simulink model "symmetric_lht"  (R2020a)
settings: Solver=FixedStepDiscrete  StartTime=0.0  StopTime=inf  RelTol=1e-3
values from neighbouring files (symbols this model uses):
  fs = fclk(1)*1e6    [setupSystem.m]
  height = heightName(nameIdx)    [setupSystem.m]
  inarray = uint8(simDirNew)    [setupSystem.m]
  nRho = maxRho*2    [setupSystem.m]
  nTheta = length(theta)    [setupSystem.m]
  theta = 0:1:179    [SymmetricLHT.m]    (also in setupSystem.m = (0:1:179))
  width = widthName(nameIdx)    [setupSystem.m]
undefined symbols (not defined in the file or in its folder): rhoBits, rhoMax
libraries: hdlsllib x35, simulink x25, dspsrcs4 x1
(part 1 of 2)
settings Model: DataTypeOverride=Off  SimulationMode=rapid-accelerator  Creator=david  LastModifiedBy=david
settings OptimizationCC: BlockReduction=off  ConditionallyExecuteInputs=off  DefaultParameterBehavior=Inlined
settings DebuggingCC: AlgebraicLoopMsg=error  SingleTaskRateTransMsg=error
settings HardwareCC: ProdBitPerPointer=32  ProdBitPerSizeT=32  ProdBitPerPtrDiffT=32  ProdLargestAtomicFloat=None  ProdIntDivRoundTo=Undefined  ProdEndianess=Unspecified  ProdWordSize=32  ProdHWDeviceType=ASIC/FPGA->ASIC/FPGA  TargetBitPerPointer=64  TargetBitPerSizeT=64  TargetBitPerPtrDiffT=64  TargetLongLongMode=on  TargetIntDivRoundTo=Zero  TargetEndianess=LittleEndian  TargetWordSize=64  TargetHWDeviceType=Custom Processor->MATLAB Host Computer  ProdEqTarget=off

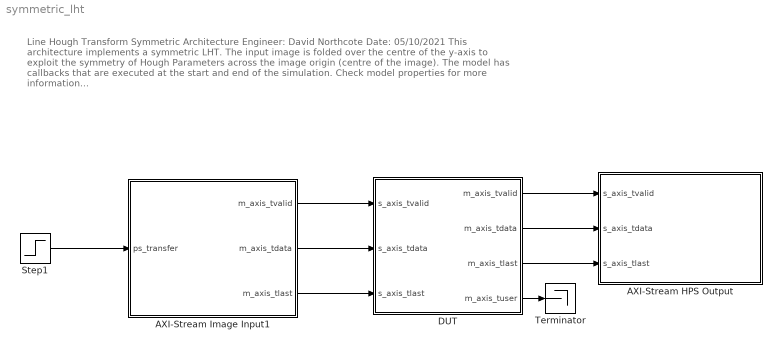
== system symmetric_lht ==
  note: Line Hough Transform Symmetric Architecture
      |
      | Engineer: David Northcote
      | Date: 05/10/2021
      |
      | This architecture implements a symmetric LHT. The input image is folded over the centre of the y-axis to exploit the symmetry of Hough Parameters across the image origin (centre of the image).
      | The model has callbacks that are executed at the start and end of the simulation. Check model properties for more information...
  AXI-Stream HPS Output : Subsystem  mask{height=nRho, width=nTheta, clk=1/fs, d=0}
      mask prompts: height "Image Height:"; width "Image Width:"; clk "Clock Rate:"; d "Frame Capture Number"
      mask DialogControl DescGroupVar Prompt: AXI-Stream Image Output
      mask DialogControl DescTextVar Prompt: Image output using the AXI-Stream interface. Simulates an AXI DMA write channel.
      mask DialogControl ParameterGroupVar Prompt: Main
  AXI-Stream Image Input1 : Subsystem  mask{image=inarray, clk=1/fs}
      mask prompts: image "Input Image:"; clk "Clock Rate:"
      mask init:
      | [height, width] = size(image);
      mask DialogControl DescGroupVar Prompt: AXI-Stream Image Input
      mask DialogControl DescTextVar Prompt: This block simulates an AXI-Stream image input for interfacing to a hardware accelerator or IP Core.
      mask DialogControl ParameterGroupVar Prompt: Main
  DUT : Subsystem  TreatAsAtomicUnit=on
  Step1 : Step  Time=2/150e6  SampleTime=1/fs
  Terminator : Terminator
  wires:
  AXI-Stream Image Input1/1(m_axis_tvalid) -> DUT/1(s_axis_tvalid)
  AXI-Stream Image Input1/2(m_axis_tdata) -> DUT/2(s_axis_tdata)
  AXI-Stream Image Input1/3(m_axis_tlast) -> DUT/3(s_axis_tlast)
  Step1/1 -> AXI-Stream Image Input1/1(ps_transfer)
  DUT/1(m_axis_tvalid) -> AXI-Stream HPS Output/1(s_axis_tvalid)
  DUT/2(m_axis_tdata) -> AXI-Stream HPS Output/2(s_axis_tdata)
  DUT/3(m_axis_tlast) -> AXI-Stream HPS Output/3(s_axis_tlast)
  DUT/4(m_axis_tuser) -> Terminator/1

== system symmetric_lht/AXI-Stream HPS Output ==
  s_axis_tvalid : Inport
  s_axis_tdata : Inport  Port=2
  s_axis_tlast : Inport  Port=3
  Delay : Delay  DelayLength=200
  Delay1 : Delay  DelayLength=d  ShowEnablePort=on
      settings: InputPortMap=u0,e6
  Pixel to Workspace : Subsystem
  Stop Simulation2 : Stop
  wires:
  s_axis_tvalid/1 -> Pixel to Workspace/Enable
  s_axis_tdata/1 -> Pixel to Workspace/1(Pixel In)
  s_axis_tlast/1 -> Delay1/2, Delay1/1
  Delay1/1 -> Delay/1
  Delay/1 -> Stop Simulation2/1

== system symmetric_lht/AXI-Stream Image Input1 ==
  ps_transfer : Inport
  Compare To Constant : simulink/Logic and Bit Operations/Compare To Constant  relop===  const=height*width-1  OutDataTypeStr=boolean
  Constant : Constant  OutDataTypeStr=boolean  SampleTime=-1
  Data Type Conversion : DataTypeConversion  OutDataTypeStr=uint32
  HDL Counter : hdlsllib/Sources/HDL Counter  CountType=Free running  CountInit=0  CountStep=1  CountMax=width*height-1  CountFromType=Initial value  CountFrom=0  CountResetPort=on  CountLoadPort=off  CountEnbPort=on  CountDirPort=off  CountDataType=Unsigned  CountWordLen=32  CountFracLen=0  CountSampTime=1
  Multiport Switch : MultiPortSwitch  DataPortOrder=Zero-based contiguous  Inputs=2  zeroidx=on
  Rising Edge Detector : Subsystem
  Synchronous Image Source : Subsystem
  Unit Delay Resettable Synchronous : hdlsllib/Discrete/Unit Delay Resettable Synchronous  InitialCondition=0.0  SampleTime=-1
      settings: SourceProductBaseCode=SL
  m_axis_tvalid : Outport
  m_axis_tdata : Outport  Port=2
  m_axis_tlast : Outport  Port=3
  wires:
  HDL Counter/1 -> Compare To Constant/1
  Synchronous Image Source/1(Pixel) -> Data Type Conversion/1
  Multiport Switch/1 -> Unit Delay Resettable Synchronous/1, HDL Counter/2, Synchronous Image Source/Enable, m_axis_tvalid/1
  Compare To Constant/1 -> Unit Delay Resettable Synchronous/2, HDL Counter/1, m_axis_tlast/1
  Data Type Conversion/1 -> m_axis_tdata/1
  ps_transfer/1 -> Rising Edge Detector/1(Input)
  Unit Delay Resettable Synchronous/1 -> Multiport Switch/2
  Rising Edge Detector/1(Output) -> Multiport Switch/1
  Constant/1 -> Multiport Switch/3

== system symmetric_lht/DUT ==
  s_axis_tvalid : Inport
  s_axis_tdata : Inport  Port=2
  s_axis_tlast : Inport  Port=3
  Symmetric Hough Accumulator : Subsystem
  Symmetric Hough Kernel : Subsystem
  m_axis_tvalid : Outport
  m_axis_tdata : Outport  Port=2
  m_axis_tlast : Outport  Port=3
  m_axis_tuser : Outport  Port=4
  wires:
  Symmetric Hough Kernel/5(EoF Out) -> Symmetric Hough Accumulator/5(EoF In)
  Symmetric Hough Kernel/6(SoF Out) -> Symmetric Hough Accumulator/6(SoF In)
  Symmetric Hough Kernel/3(Valid Out) -> Symmetric Hough Accumulator/3(Valid In)
  Symmetric Hough Kernel/2(Edge Out A) -> Symmetric Hough Accumulator/2(Edge In A)
  Symmetric Hough Kernel/4(Hough Parameters) -> Symmetric Hough Accumulator/4(HP In)
  Symmetric Hough Kernel/1(Edge Out B) -> Symmetric Hough Accumulator/1(Edge In B)
  s_axis_tvalid/1 -> Symmetric Hough Kernel/1(Valid In)
  s_axis_tdata/1 -> Symmetric Hough Kernel/2(Edge In)
  s_axis_tlast/1 -> Symmetric Hough Kernel/3(EoF In)
  Symmetric Hough Accumulator/1(Valid Out) -> m_axis_tvalid/1
  Symmetric Hough Accumulator/2(HP Out) -> m_axis_tdata/1
  Symmetric Hough Accumulator/3(EoF Out) -> m_axis_tlast/1
  Symmetric Hough Accumulator/4(SoF Out) -> m_axis_tuser/1

== system symmetric_lht/AXI-Stream HPS Output/Pixel to Workspace ==
  Pixel In : Inport
  Enable : EnablePort
  To Workspace : ToWorkspace  VariableName=simout  SampleTime=-1
      settings: MaxDataPoints=height*width  Save2DSignal=2-D array (concatenate along first dimension)
  wires:
  Pixel In/1 -> To Workspace/1

== system symmetric_lht/AXI-Stream Image Input1/Rising Edge Detector ==
  Input : Inport
  AND : Logic  IconShape=distinctive  AllPortsSameDT=off  OutDataTypeStr=boolean
  Delay : Delay  DelayLength=1
  NOT : Logic  Operator=NOT  IconShape=distinctive  AllPortsSameDT=off  OutDataTypeStr=boolean
  Output : Outport  VectorParamsAs1DForOutWhenUnconnected=off
  wires:
  NOT/1 -> Delay/1
  Input/1 -> AND/2, NOT/1
  Delay/1 -> AND/1
  AND/1 -> Output/1

== system symmetric_lht/AXI-Stream Image Input1/Synchronous Image Source ==
  Enable : EnablePort
  Signal From Workspace : dspsrcs4/Signal From Workspace  X=reshape(image', [height*width, 1])  Ts=clk  nsamps=1  OutputAfterFinalValue=Cyclic repetition  ignoreOrWarnInputAndFrameLengths=off  OutputFrames=off
  Pixel : Outport
  wires:
  Signal From Workspace/1 -> Pixel/1

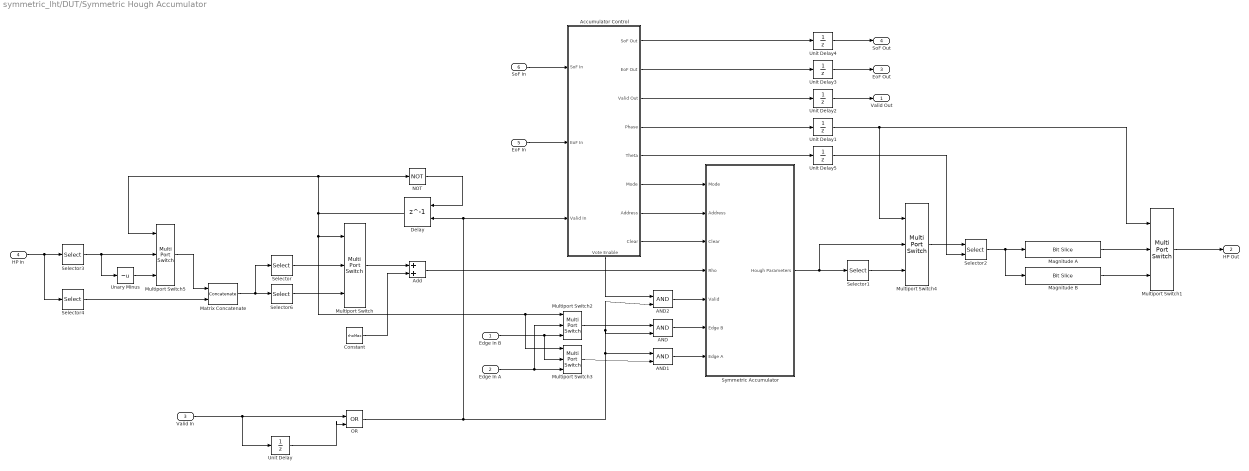
== system symmetric_lht/DUT/Symmetric Hough Accumulator ==
  Edge In B : Inport
  Edge In A : Inport  Port=2
  Valid In : Inport  Port=3
  HP In : Inport  Port=4
  EoF In : Inport  Port=5
  SoF In : Inport  Port=6
  AND : Logic  IconShape=distinctive  AllPortsSameDT=off  OutDataTypeStr=boolean
  AND1 : Logic  IconShape=distinctive  AllPortsSameDT=off  OutDataTypeStr=boolean
  AND2 : Logic  IconShape=distinctive  AllPortsSameDT=off  OutDataTypeStr=boolean
  Accumulator Control : Subsystem
      settings: PortSchema="{\"entries\":[{\"content\":{\"sides\":[{\"content\":{\"connectorIds\":[\"In1\",\"In2\",\"In3\"]},\"type\":\"ConnectorPlacement.EquallySpacedRectSide\",\"uuid\":\"a55fcade-e911-4d62-bb2d-85c447a0f5bf\"},{\"content\":{\"connectorIds\":[\"Out1\",\"Out2\",\"Out3\",\"Out4\",\"Out5\",\"Out6\",\"Out7\",\"Out8\"],\"side\":\"RIGHT\"},\"type\":\"ConnectorPlacement.EquallySpacedRectSide\",\"uuid\":\"4fd7641f-084e-41b1-b176-c069ded5b82c\"},{\"content\":{\"connectorIds\":[],\"side\":\"TOP\"},\"type\":\"ConnectorPlacement.EquallySpacedRectSide\",\"uuid\":\"deed3939-6347-4cb7-b219-ca9c7d26ba03\"},{\"content\":{\"connectorIds\":[\"Out9\"],\"side\":\"BOTTOM\"},\"type\":\"ConnectorPlacement.EquallySpacedRectSide\",\"uuid\":\"54e68855-cbe1-4376-a294-01ca31feaad6\"}]},\"type\":\"ConnectorPlacement.EquallySpacedConnector\",\"uuid\":\"189d7daa-73d7-445a-9112-0e847ff32020\"}],\"packageUris\":[\"http://schema.mathworks.com/mf0/Connector/19700101\"],\"version\":\"1.0\"}"
  Add : Sum  OutDataTypeStr=fixdt(0, ceil(log2(rhoMax*2)),0)
  Constant : Constant  Value=rhoMax  OutDataTypeStr=fixdt(0, ceil(log2(rhoMax+1)), 0)  SampleTime=-1
  Delay : Delay  DelayLength=1  ShowEnablePort=on
      settings: InputPortMap=u0,e6
  Magnitude A : hdlsllib/Logic and Bit Operations/Bit Slice  lidx=rhoBits-1  ridx=0
      settings: SourceProductBaseCode=SL
  Magnitude B : hdlsllib/Logic and Bit Operations/Bit Slice  lidx=rhoBits*2-1  ridx=rhoBits
      settings: SourceProductBaseCode=SL
  Matrix Concatenate : Concatenate  Mode=Multidimensional array  ConcatenateDimension=2
  Multiport Switch{,1..5} (6 alike) : MultiPortSwitch  DataPortOrder=Zero-based contiguous  Inputs=2  zeroidx=on
  NOT : Logic  Operator=NOT  IconShape=distinctive  AllPortsSameDT=off  OutDataTypeStr=boolean
  OR : Logic  Operator=OR  IconShape=distinctive  AllPortsSameDT=off  OutDataTypeStr=boolean
  Selector : Selector  IndexMode=Zero-based  InputPortWidth=180  IndexOptions=Index vector (dialog)  Indices=[0:1:length(theta)/2]  OutputSizes=1
  Selector1 : Selector  NumberOfDimensions=2  IndexMode=Zero-based  InputPortWidth=3  IndexOptions=Index vector (dialog),Index vector (dialog)  Indices=0,[0, length(theta)/2-1:-1:1]  OutputSizes=1,1
  Selector2 : Selector  NumberOfDimensions=2  IndexMode=Zero-based  InputPortWidth=length(theta)/2  IndexOptions=Index vector (dialog),Index vector (port)  Indices=0,0  OutputSizes=1,1
  Selector3 : Selector  NumberOfDimensions=2  IndexMode=Zero-based  InputPortWidth=180  IndexOptions=Index vector (dialog),Index vector (dialog)  Indices=0,0  OutputSizes=1,1
  Selector4 : Selector  NumberOfDimensions=2  IndexMode=Zero-based  InputPortWidth=180  IndexOptions=Index vector (dialog),Index vector (dialog)  Indices=0,1:1:length(theta)-1  OutputSizes=1,1
  Selector6 : Selector  IndexMode=Zero-based  InputPortWidth=180  IndexOptions=Index vector (dialog)  Indices=[0, length(theta)-1:-1:length(theta)/2]  OutputSizes=1
  Symmetric Accumulator : Subsystem
  Unary Minus : UnaryMinus
  Unit Delay{,1..5} (6 alike) : UnitDelay  SampleTime=-1  HasFrameUpgradeWarning=on
  Valid Out : Outport
  HP Out : Outport  Port=2
  EoF Out : Outport  Port=3
  SoF Out : Outport  Port=4
  wires:
  Selector4/1 -> Matrix Concatenate/2
  Unary Minus/1 -> Multiport Switch5/3
  Selector3/1 -> Multiport Switch5/2, Unary Minus/1
  Multiport Switch5/1 -> Matrix Concatenate/1
  Matrix Concatenate/1 -> Selector6/1, Selector/1
  HP In/1 -> Selector3/1, Selector4/1
  Selector1/1 -> Multiport Switch4/3
  Symmetric Accumulator/1(Hough Parameters) -> Selector1/1, Multiport Switch4/2
  Selector2/1 -> Magnitude A/1, Magnitude B/1
  Multiport Switch4/1 -> Selector2/1
  EoF In/1 -> Accumulator Control/2(EoF In)
  Multiport Switch3/1 -> AND1/2
  Edge In B/1 -> Multiport Switch3/2, Multiport Switch2/3
  Edge In A/1 -> Multiport Switch2/2, Multiport Switch3/3
  Selector6/1 -> Multiport Switch/3
  Multiport Switch2/1 -> AND/1
  Multiport Switch1/1 -> HP Out/1
  Magnitude B/1 -> Multiport Switch1/3
  Magnitude A/1 -> Multiport Switch1/2
  Constant/1 -> Add/2
  Add/1 -> Symmetric Accumulator/4(Rho)
  Multiport Switch/1 -> Add/1
  Accumulator Control/8(Clear) -> Symmetric Accumulator/3(Clear)
  Unit Delay1/1 -> Multiport Switch4/1, Multiport Switch1/1
  Unit Delay5/1 -> Selector2/2
  Accumulator Control/5(Theta) -> Unit Delay5/1
  Accumulator Control/9(Vote Enable) -> AND2/1
  AND2/1 -> Symmetric Accumulator/5(Valid)
  Accumulator Control/1(SoF Out) -> Unit Delay4/1
  Unit Delay4/1 -> SoF Out/1
  Unit Delay3/1 -> EoF Out/1
  Accumulator Control/2(EoF Out) -> Unit Delay3/1
  SoF In/1 -> Accumulator Control/1(SoF In)
  Accumulator Control/7(Address) -> Symmetric Accumulator/2(Address)
  Accumulator Control/6(Mode) -> Symmetric Accumulator/1(Mode)
  Accumulator Control/4(Phase) -> Unit Delay1/1
  Accumulator Control/3(Valid Out) -> Unit Delay2/1
  Unit Delay2/1 -> Valid Out/1
  Selector/1 -> Multiport Switch/2
  Delay/1 -> Multiport Switch2/1, Multiport Switch3/1, Multiport Switch/1, NOT/1, Multiport Switch5/1
  AND1/1 -> Symmetric Accumulator/7(Edge A)
  AND/1 -> Symmetric Accumulator/6(Edge B)
  OR/1 -> AND1/1, AND/2, AND2/2, Accumulator Control/3(Valid In), Delay/2
  Valid In/1 -> Unit Delay/1, OR/1
  Unit Delay/1 -> OR/2
  NOT/1 -> Delay/1

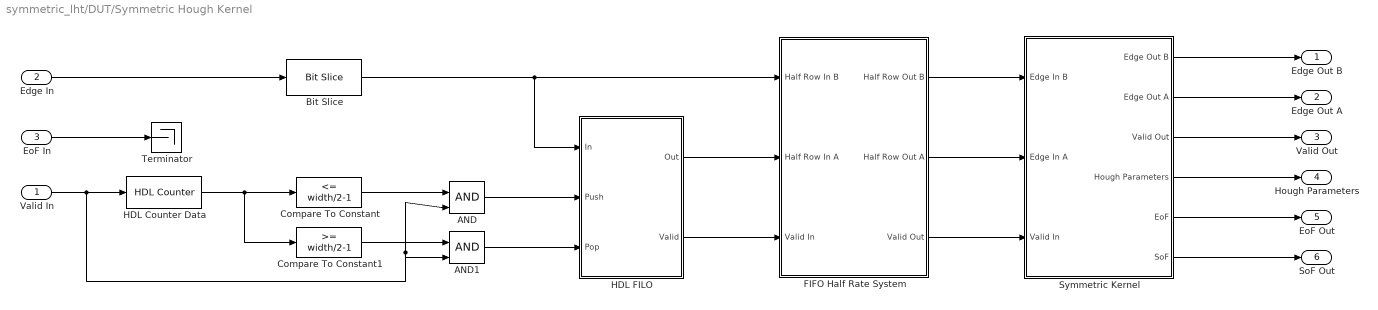
== system symmetric_lht/DUT/Symmetric Hough Kernel ==
  Valid In : Inport
  Edge In : Inport  Port=2
  EoF In : Inport  Port=3
  AND : Logic  IconShape=distinctive  AllPortsSameDT=off  OutDataTypeStr=boolean
  AND1 : Logic  IconShape=distinctive  AllPortsSameDT=off  OutDataTypeStr=boolean
  Bit Slice : hdlsllib/Logic and Bit Operations/Bit Slice  lidx=0  ridx=0
      settings: SourceProductBaseCode=SL
  Compare To Constant : simulink/Logic and Bit Operations/Compare To Constant  relop=<=  const=width/2-1  OutDataTypeStr=boolean
  Compare To Constant1 : simulink/Logic and Bit Operations/Compare To Constant  relop=>=  const=width/2-1  OutDataTypeStr=boolean
  FIFO Half Rate System : Subsystem
  HDL Counter Data : hdlsllib/Sources/HDL Counter  CountType=Count limited  CountInit=0  CountStep=1  CountMax=width-1  CountFromType=Initial value  CountFrom=0  CountResetPort=off  CountLoadPort=off  CountEnbPort=on  CountDirPort=off  CountDataType=Unsigned  CountWordLen=ceil(log2(width))  CountFracLen=0  CountSampTime=1/fs
  HDL FILO : Subsystem  mask{size=width/2}
      mask prompts: size "Register size:"
      mask DialogControl DescGroupVar Prompt: HDL FILO
      mask DialogControl DescTextVar Prompt: Implements a synchronous "First In, Last Out" (FILO) register.
  Symmetric Kernel : Subsystem
  Terminator : Terminator
  Edge Out B : Outport
  Edge Out A : Outport  Port=2
  Valid Out : Outport  Port=3
  Hough Parameters : Outport  Port=4
  EoF Out : Outport  Port=5
  SoF Out : Outport  Port=6
  wires:
  HDL Counter Data/1 -> Compare To Constant1/1, Compare To Constant/1
  Edge In/1 -> Bit Slice/1
  Symmetric Kernel/1(Edge Out B) -> Edge Out B/1
  HDL FILO/1(Out) -> FIFO Half Rate System/2(Half Row In A)
  FIFO Half Rate System/1(Half Row Out B) -> Symmetric Kernel/1(Edge In B)
  Valid In/1 -> AND/2, AND1/2, HDL Counter Data/1
  FIFO Half Rate System/2(Half Row Out A) -> Symmetric Kernel/2(Edge In A)
  HDL FILO/2(Valid) -> FIFO Half Rate System/3(Valid In)
  FIFO Half Rate System/3(Valid Out) -> Symmetric Kernel/3(Valid In)
  Symmetric Kernel/3(Valid Out) -> Valid Out/1
  Symmetric Kernel/4(Hough Parameters) -> Hough Parameters/1
  Symmetric Kernel/5(EoF) -> EoF Out/1
  Symmetric Kernel/2(Edge Out A) -> Edge Out A/1
  EoF In/1 -> Terminator/1
  Compare To Constant/1 -> AND/1
  AND/1 -> HDL FILO/2(Push)
  AND1/1 -> HDL FILO/3(Pop)
  Compare To Constant1/1 -> AND1/1
  Symmetric Kernel/6(SoF) -> SoF Out/1
  Bit Slice/1 -> HDL FILO/1(In), FIFO Half Rate System/1(Half Row In B)

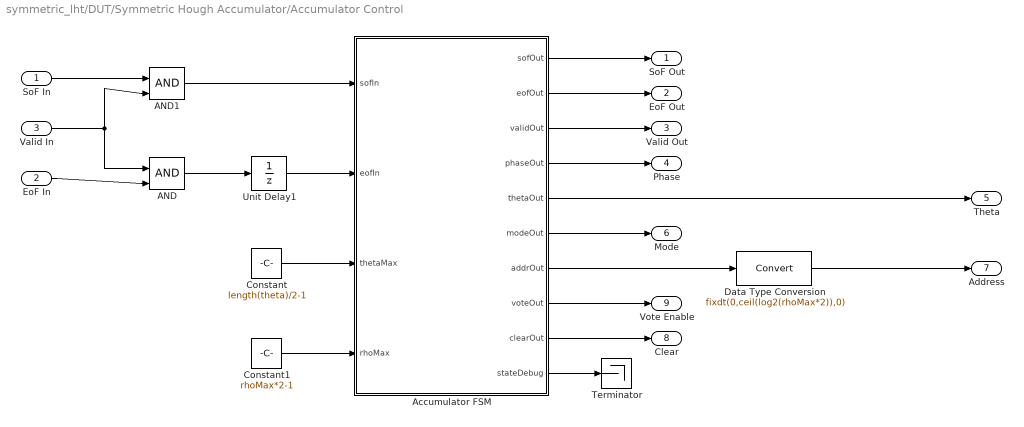
== system symmetric_lht/DUT/Symmetric Hough Accumulator/Accumulator Control ==
  SoF In : Inport
  EoF In : Inport  Port=2
  Valid In : Inport  Port=3
  AND : Logic  IconShape=distinctive  AllPortsSameDT=off  OutDataTypeStr=boolean
  AND1 : Logic  IconShape=distinctive  AllPortsSameDT=off  OutDataTypeStr=boolean
  Accumulator FSM : MATLAB Function  TreatAsAtomicUnit=on
  Constant : Constant  Value=length(theta)/2-1  OutDataTypeStr=uint8  SampleTime=-1
  Constant1 : Constant  Value=rhoMax*2-1  OutDataTypeStr=uint16  SampleTime=-1
  Data Type Conversion : DataTypeConversion  OutDataTypeStr=fixdt(0,ceil(log2(rhoMax*2)),0)
  Terminator : Terminator
  Unit Delay1 : UnitDelay  SampleTime=-1  HasFrameUpgradeWarning=on
  SoF Out : Outport
  EoF Out : Outport  Port=2
  Valid Out : Outport  Port=3
  Phase : Outport  Port=4
  Theta : Outport  Port=5
  Mode : Outport  Port=6
  Address : Outport  Port=7
  Clear : Outport  Port=8
  Vote Enable : Outport  Port=9
  wires:
  Unit Delay1/1 -> Accumulator FSM/2(eofIn)
  AND/1 -> Unit Delay1/1
  Accumulator FSM/5(thetaOut) -> Theta/1
  Accumulator FSM/9(clearOut) -> Clear/1
  Data Type Conversion/1 -> Address/1
  Accumulator FSM/10(stateDebug) -> Terminator/1
  Constant1/1 -> Accumulator FSM/4(rhoMax)
  Constant/1 -> Accumulator FSM/3(thetaMax)
  Accumulator FSM/8(voteOut) -> Vote Enable/1
  Accumulator FSM/7(addrOut) -> Data Type Conversion/1
  Accumulator FSM/6(modeOut) -> Mode/1
  Accumulator FSM/4(phaseOut) -> Phase/1
  Accumulator FSM/3(validOut) -> Valid Out/1
  Accumulator FSM/2(eofOut) -> EoF Out/1
  Accumulator FSM/1(sofOut) -> SoF Out/1
  AND1/1 -> Accumulator FSM/1(sofIn)
  EoF In/1 -> AND/2
  Valid In/1 -> AND/1, AND1/2
  SoF In/1 -> AND1/1

== system symmetric_lht/DUT/Symmetric Hough Accumulator/Symmetric Accumulator ==
  Mode : Inport
  Address : Inport  Port=2
  Clear : Inport  Port=3
  Rho : Inport  Port=4
  Valid : Inport  Port=5
  Edge B : Inport  Port=6
  Edge A : Inport  Port=7
  Bit Concat : hdlsllib/Logic and Bit Operations/Bit Concat  numInputs=2
  First Phase Memory : Subsystem
  Matrix Concatenate : Concatenate  Mode=Multidimensional array  ConcatenateDimension=2
  Second Phase Memory : Subsystem
  Selector : Selector  NumberOfDimensions=2  IndexMode=Zero-based  InputPortWidth=3  IndexOptions=Index vector (dialog),Index vector (dialog)  Indices=0,0  OutputSizes=1,1
  Selector1 : Selector  NumberOfDimensions=2  IndexMode=Zero-based  InputPortWidth=3  IndexOptions=Index vector (dialog),Index vector (dialog)  Indices=0,1:1:length(theta)/2-1  OutputSizes=1,1
  Selector2 : Selector  NumberOfDimensions=2  IndexMode=Zero-based  InputPortWidth=3  IndexOptions=Index vector (dialog),Index vector (dialog)  Indices=0,length(theta)/2  OutputSizes=1,1
  Symmetric Memory : Subsystem
  Hough Parameters : Outport
  wires:
  Selector/1 -> First Phase Memory/4(Rho)
  Selector2/1 -> Second Phase Memory/4(Rho)
  Second Phase Memory/1(Hough Parameters) -> Bit Concat/1
  First Phase Memory/1(Hough Parameters) -> Bit Concat/2
  Edge B/1 -> Symmetric Memory/6(Edge B), Second Phase Memory/6(Edge)
  Bit Concat/1 -> Matrix Concatenate/1
  Symmetric Memory/1(Hough Parameters) -> Matrix Concatenate/2
  Selector1/1 -> Symmetric Memory/4(Rho)
  Matrix Concatenate/1 -> Hough Parameters/1
  Edge A/1 -> Symmetric Memory/7(Edge A), First Phase Memory/6(Edge)
  Valid/1 -> Second Phase Memory/5(Valid), First Phase Memory/5(Valid), Symmetric Memory/5(Valid)
  Rho/1 -> Selector1/1, Selector/1, Selector2/1
  Clear/1 -> Symmetric Memory/3(Clear), First Phase Memory/3(Clear), Second Phase Memory/3(Clear)
  Address/1 -> Symmetric Memory/2(Address), First Phase Memory/2(Address), Second Phase Memory/2(Address)
  Mode/1 -> Symmetric Memory/1(Mode), First Phase Memory/1(Mode), Second Phase Memory/1(Mode)

== system symmetric_lht/DUT/Symmetric Hough Kernel/FIFO Half Rate System ==
  Half Row In B : Inport
  Half Row In A : Inport  Port=2
  Valid In : Inport  Port=3
  FIFO Half Rate A : Subsystem
  FIFO Half Rate B : Subsystem
  Terminator : Terminator
  Half Row Out B : Outport
  Half Row Out A : Outport  Port=2
  Valid Out : Outport  Port=3
  wires:
  FIFO Half Rate B/1(Out) -> Half Row Out B/1
  Half Row In B/1 -> FIFO Half Rate B/1(In)
  Valid In/1 -> FIFO Half Rate A/2(Push), FIFO Half Rate B/2(Push)
  FIFO Half Rate B/2(Valid) -> Terminator/1
  FIFO Half Rate A/1(Out) -> Half Row Out A/1
  Half Row In A/1 -> FIFO Half Rate A/1(In)
  FIFO Half Rate A/2(Valid) -> Valid Out/1

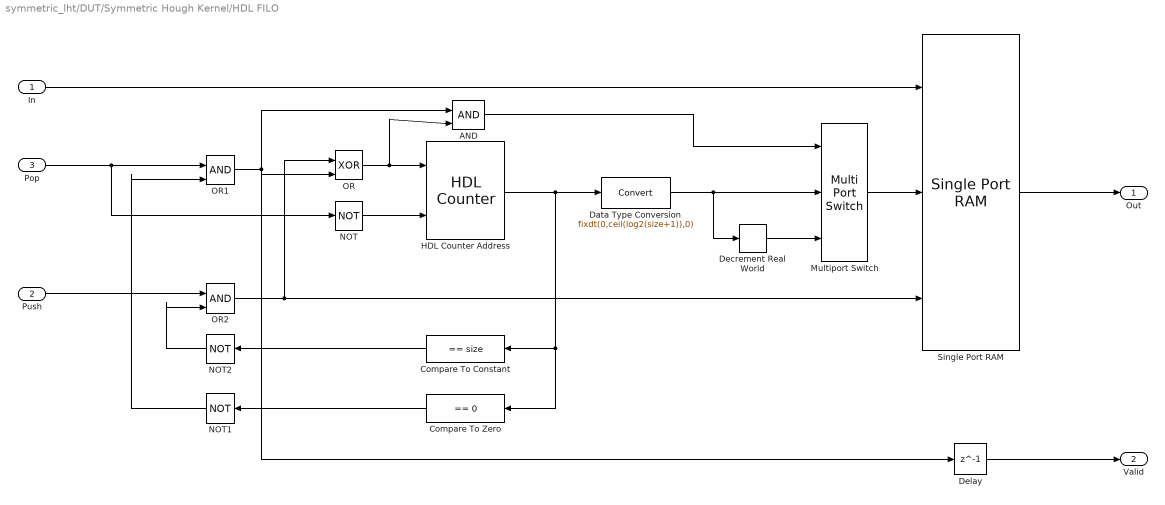
== system symmetric_lht/DUT/Symmetric Hough Kernel/HDL FILO ==
  In : Inport
  Push : Inport  Port=2
  Pop : Inport  Port=3
  AND : Logic  IconShape=distinctive  AllPortsSameDT=off  OutDataTypeStr=boolean
  Compare To Constant : simulink/Logic and Bit Operations/Compare To Constant  relop===  const=size  OutDataTypeStr=boolean
  Compare To Zero : simulink/Logic and Bit Operations/Compare To Zero  relop===  OutDataTypeStr=boolean
  Data Type Conversion : DataTypeConversion  OutDataTypeStr=fixdt(0,ceil(log2(size+1)),0)
  Decrement Real World : simulink/Additional Math & Discrete/Additional Math: Increment - Decrement/Decrement Real World
      settings: SourceProductBaseCode=SL
  Delay : Delay  DelayLength=1
  HDL Counter Address : hdlsllib/Sources/HDL Counter  CountType=Count limited  CountInit=0  CountStep=1  CountMax=size+1  CountFromType=Initial value  CountFrom=0  CountResetPort=off  CountLoadPort=off  CountEnbPort=on  CountDirPort=on  CountDataType=Unsigned  CountWordLen=ceil(log2(size+2))  CountFracLen=0  CountSampTime=1
  Multiport Switch : MultiPortSwitch  DataPortOrder=Zero-based contiguous  Inputs=2  zeroidx=on
  NOT : Logic  Operator=NOT  IconShape=distinctive  AllPortsSameDT=off  OutDataTypeStr=boolean
  NOT1 : Logic  Operator=NOT  IconShape=distinctive  AllPortsSameDT=off  OutDataTypeStr=boolean
  NOT2 : Logic  Operator=NOT  IconShape=distinctive  AllPortsSameDT=off  OutDataTypeStr=boolean
  OR : Logic  Operator=XOR  IconShape=distinctive  AllPortsSameDT=off  OutDataTypeStr=boolean
  OR1 : Logic  IconShape=distinctive  AllPortsSameDT=off  OutDataTypeStr=boolean
  OR2 : Logic  IconShape=distinctive  AllPortsSameDT=off  OutDataTypeStr=boolean
  Single Port RAM : hdlsllib/HDL RAMs/Single Port RAM  ram_size=ceil(log2(size+1))  dout_type=New data
      settings: SourceProductBaseCode=SL
  Out : Outport
  Valid : Outport  Port=2
  wires:
  NOT/1 -> HDL Counter Address/2
  Data Type Conversion/1 -> Decrement Real World/1, Multiport Switch/2
  Decrement Real World/1 -> Multiport Switch/3
  Multiport Switch/1 -> Single Port RAM/2
  HDL Counter Address/1 -> Data Type Conversion/1, Compare To Zero/1, Compare To Constant/1
  Compare To Constant/1 -> NOT2/1
  NOT2/1 -> OR2/2
  NOT1/1 -> OR1/2
  Compare To Zero/1 -> NOT1/1
  In/1 -> Single Port RAM/1
  Push/1 -> OR2/1
  Single Port RAM/1 -> Out/1
  OR/1 -> AND/2, HDL Counter Address/1
  OR1/1 -> Delay/1, AND/1, OR/2
  Pop/1 -> NOT/1, OR1/1
  OR2/1 -> Single Port RAM/3, OR/1
  Delay/1 -> Valid/1
  AND/1 -> Multiport Switch/1

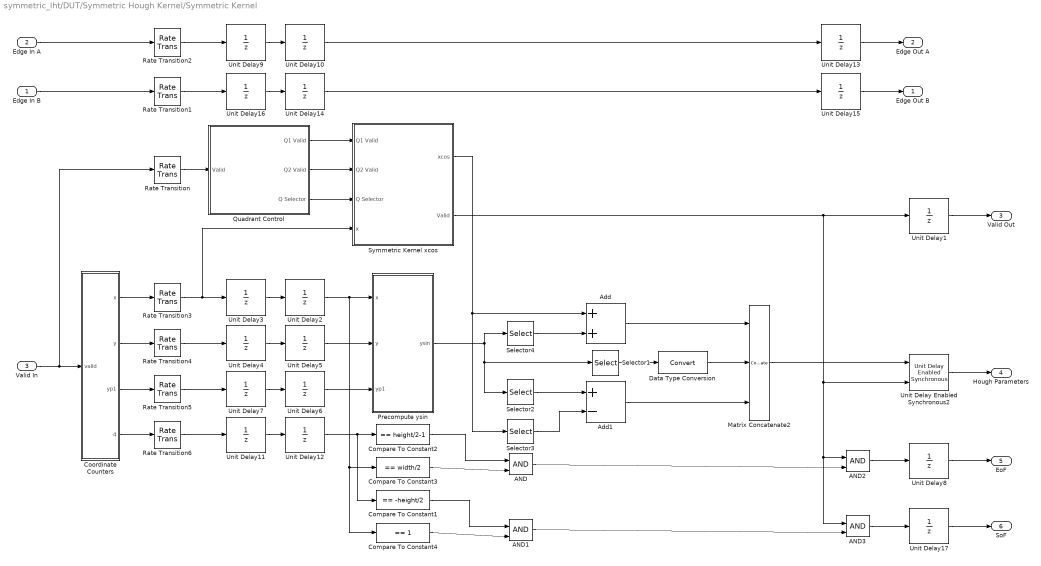
== system symmetric_lht/DUT/Symmetric Hough Kernel/Symmetric Kernel ==
  Edge In B : Inport
  Edge In A : Inport  Port=2
  Valid In : Inport  Port=3
  AND{,1..3} (4 alike) : Logic  IconShape=distinctive  AllPortsSameDT=off  OutDataTypeStr=boolean
  Add : Sum  OutDataTypeStr=fixdt(1,ceil(log2(rhoMax*2)),0)  RndMeth=Round  SaturateOnIntegerOverflow=on
  Add1 : Sum  Inputs=+-  OutDataTypeStr=fixdt(1, ceil(log2(2*rhoMax)), 0)  RndMeth=Round  SaturateOnIntegerOverflow=on
  Compare To Constant1 : simulink/Logic and Bit Operations/Compare To Constant  relop===  const=-height/2  OutDataTypeStr=boolean
  Compare To Constant2 : simulink/Logic and Bit Operations/Compare To Constant  relop===  const=height/2-1  OutDataTypeStr=boolean
  Compare To Constant3 : simulink/Logic and Bit Operations/Compare To Constant  relop===  const=width/2  OutDataTypeStr=boolean
  Compare To Constant4 : simulink/Logic and Bit Operations/Compare To Constant  relop===  const=1  OutDataTypeStr=boolean
  Coordinate Counters : Subsystem
  Data Type Conversion : DataTypeConversion
  Matrix Concatenate2 : Concatenate  NumInputs=3  Mode=Multidimensional array  ConcatenateDimension=2
  Precompute ysin : Subsystem
  Quadrant Control : Subsystem
  Rate Transition : RateTransition
  Rate Transition1 : RateTransition
  Rate Transition2 : RateTransition
  Rate Transition{3..6} (4 alike) : RateTransition  OutPortSampleTimeOpt=Multiple of input port sample time  OutPortSampleTimeMultiple=1/2
  Selector1 : Selector  InputPortWidth=91  IndexOptions=Index vector (dialog)  Indices=91  OutputSizes=1
  Selector2 : Selector  InputPortWidth=91  IndexOptions=Index vector (dialog)  Indices=[90:-1:2]  OutputSizes=1
  Selector3 : Selector  InputPortWidth=90  IndexOptions=Index vector (dialog)  Indices=[90:-1:2]  OutputSizes=1
  Selector4 : Selector  InputPortWidth=91  IndexOptions=Index vector (dialog)  Indices=[1:1:90]  OutputSizes=1
  Symmetric Kernel xcos : Subsystem
  Unit Delay Enabled Synchronous2 : hdlsllib/Discrete/Unit Delay Enabled Synchronous  InitialCondition=0.0  SampleTime=-1
      settings: SourceProductBaseCode=SL
  Unit Delay{1..17} (17 alike) : UnitDelay  SampleTime=-1  HasFrameUpgradeWarning=on
  Edge Out B : Outport
  Edge Out A : Outport  Port=2
  Valid Out : Outport  Port=3
  Hough Parameters : Outport  Port=4
  EoF : Outport  Port=5
  SoF : Outport  Port=6
  wires:
  Unit Delay8/1 -> EoF/1
  Quadrant Control/3(Q Selector) -> Symmetric Kernel xcos/3(Q Selector)
  Add/1 -> Matrix Concatenate2/1
  Quadrant Control/2(Q2 Valid) -> Symmetric Kernel xcos/2(Q2 Valid)
  Coordinate Counters/3(yp1) -> Rate Transition5/1
  Rate Transition5/1 -> Unit Delay7/1
  Unit Delay7/1 -> Unit Delay6/1
  Symmetric Kernel xcos/2(Valid) -> Unit Delay1/1, AND3/1, AND2/1, Unit Delay Enabled Synchronous2/2
  Valid In/1 -> Rate Transition/1, Coordinate Counters/1(valid)
  Rate Transition4/1 -> Unit Delay4/1
  Quadrant Control/1(Q1 Valid) -> Symmetric Kernel xcos/1(Q1 Valid)
  Unit Delay3/1 -> Unit Delay2/1
  Unit Delay11/1 -> Unit Delay12/1
  Unit Delay Enabled Synchronous2/1 -> Hough Parameters/1
  Precompute ysin/1(ysin) -> Selector1/1, Selector2/1, Selector4/1
  Unit Delay4/1 -> Unit Delay5/1
  Coordinate Counters/2(y) -> Rate Transition4/1
  Rate Transition6/1 -> Unit Delay11/1
  Unit Delay12/1 -> Compare To Constant1/1, Compare To Constant2/1
  Coordinate Counters/1(x) -> Rate Transition3/1
  Unit Delay1/1 -> Valid Out/1
  Selector2/1 -> Add1/1
  Unit Delay2/1 -> Precompute ysin/1(x), Compare To Constant4/1, Compare To Constant3/1
  Rate Transition3/1 -> Symmetric Kernel xcos/4(x), Unit Delay3/1
  Unit Delay6/1 -> Precompute ysin/3(yp1)
  Unit Delay5/1 -> Precompute ysin/2(y)
  Compare To Constant2/1 -> AND/1
  Matrix Concatenate2/1 -> Unit Delay Enabled Synchronous2/1
  Compare To Constant3/1 -> AND/2
  Selector3/1 -> Add1/2
  Coordinate Counters/4(y relative) -> Rate Transition6/1
  Edge In A/1 -> Rate Transition2/1
  Rate Transition2/1 -> Unit Delay9/1
  Unit Delay9/1 -> Unit Delay10/1
  Unit Delay10/1 -> Unit Delay13/1
  Unit Delay13/1 -> Edge Out A/1
  Unit Delay15/1 -> Edge Out B/1
  Unit Delay14/1 -> Unit Delay15/1
  Unit Delay16/1 -> Unit Delay14/1
  Rate Transition1/1 -> Unit Delay16/1
  Edge In B/1 -> Rate Transition1/1
  Rate Transition/1 -> Quadrant Control/1(Valid)
  Compare To Constant4/1 -> AND1/2
  Compare To Constant1/1 -> AND1/1
  Unit Delay17/1 -> SoF/1
  AND2/1 -> Unit Delay8/1
  AND/1 -> AND2/2
  AND3/1 -> Unit Delay17/1
  AND1/1 -> AND3/2
  Add1/1 -> Matrix Concatenate2/3
  Selector1/1 -> Data Type Conversion/1
  Selector4/1 -> Add/2
  Symmetric Kernel xcos/1(xcos) -> Add/1, Selector3/1
  Data Type Conversion/1 -> Matrix Concatenate2/2

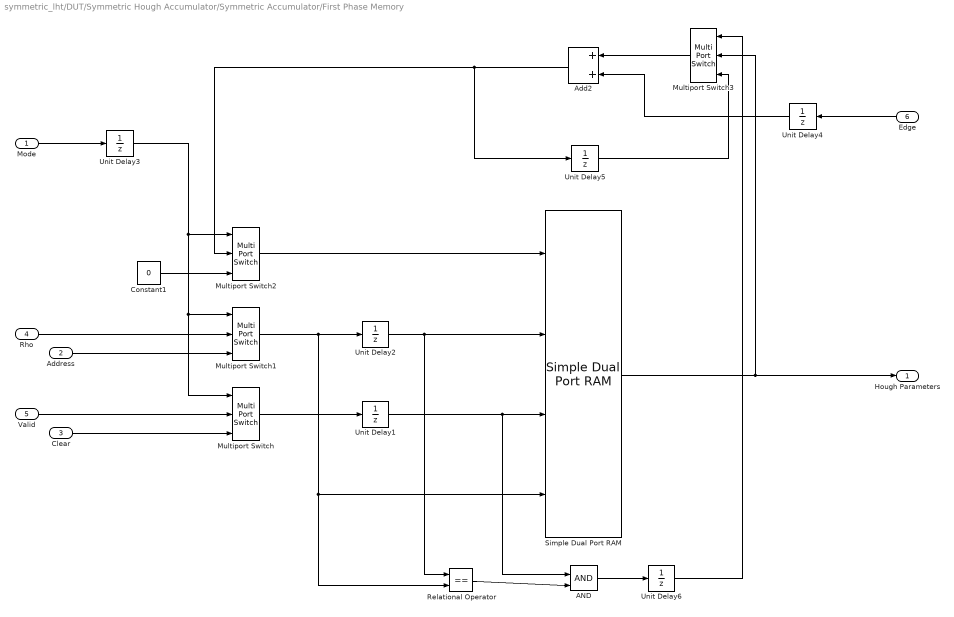
== system symmetric_lht/DUT/Symmetric Hough Accumulator/Symmetric Accumulator/First Phase Memory ==
  Mode : Inport
  Address : Inport  Port=2
  Clear : Inport  Port=3
  Rho : Inport  Port=4
  Valid : Inport  Port=5
  Edge : Inport  Port=6
  AND : Logic  IconShape=distinctive  AllPortsSameDT=off  OutDataTypeStr=boolean
  Add2 : Sum  OutDataTypeStr=Inherit: Same as first input
  Constant1 : Constant  Value=0  OutDataTypeStr=fixdt(0,rhoBits,0)  SampleTime=-1
  Multiport Switch{,1..3} (4 alike) : MultiPortSwitch  DataPortOrder=Zero-based contiguous  Inputs=2  zeroidx=on
  Relational Operator : RelationalOperator  Operator===  OutDataTypeStr=boolean  RndMeth=Simplest
  Simple Dual Port RAM : hdlsllib/HDL RAMs/Simple Dual Port RAM  ram_size=ceil(log2(rhoMax*2))
      settings: SourceProductBaseCode=SL
  Unit Delay{1..6} (6 alike) : UnitDelay  SampleTime=-1  HasFrameUpgradeWarning=on
  Hough Parameters : Outport
  wires:
  Unit Delay4/1 -> Add2/2
  Multiport Switch3/1 -> Add2/1
  Relational Operator/1 -> AND/2
  Unit Delay6/1 -> Multiport Switch3/1
  AND/1 -> Unit Delay6/1
  Unit Delay5/1 -> Multiport Switch3/3
  Simple Dual Port RAM/1 -> Hough Parameters/1, Multiport Switch3/2
  Add2/1 -> Multiport Switch2/2, Unit Delay5/1
  Multiport Switch1/1 -> Simple Dual Port RAM/4, Relational Operator/2, Unit Delay2/1
  Edge/1 -> Unit Delay4/1
  Address/1 -> Multiport Switch1/3
  Mode/1 -> Unit Delay3/1
  Multiport Switch/1 -> Unit Delay1/1
  Multiport Switch2/1 -> Simple Dual Port RAM/1
  Unit Delay3/1 -> Multiport Switch2/1, Multiport Switch1/1, Multiport Switch/1
  Clear/1 -> Multiport Switch/3
  Rho/1 -> Multiport Switch1/2
  Unit Delay1/1 -> Simple Dual Port RAM/3, AND/1
  Unit Delay2/1 -> Simple Dual Port RAM/2, Relational Operator/1
  Constant1/1 -> Multiport Switch2/3
  Valid/1 -> Multiport Switch/2

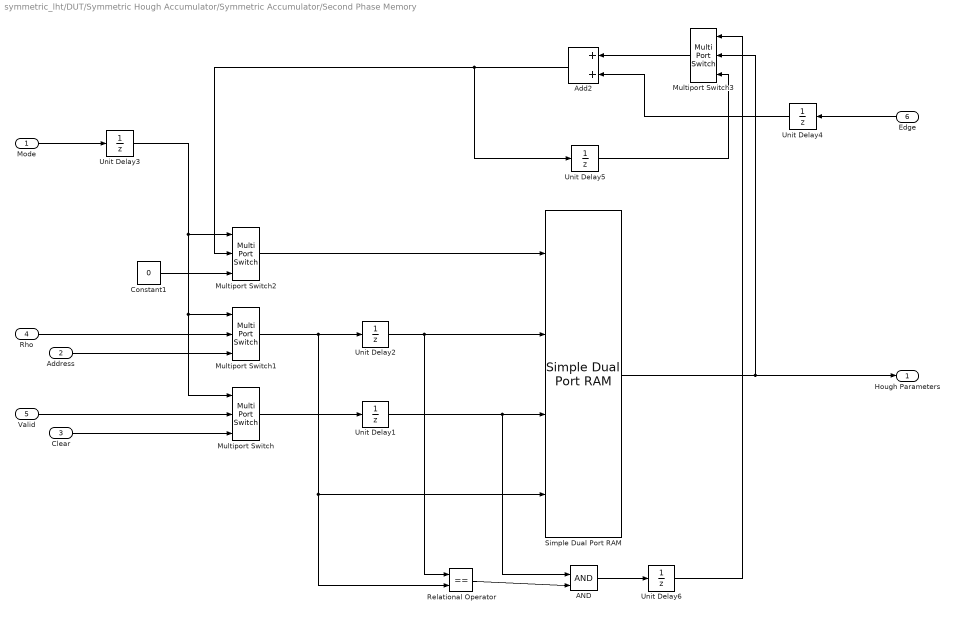
== system symmetric_lht/DUT/Symmetric Hough Accumulator/Symmetric Accumulator/Second Phase Memory ==
  Mode : Inport
  Address : Inport  Port=2
  Clear : Inport  Port=3
  Rho : Inport  Port=4
  Valid : Inport  Port=5
  Edge : Inport  Port=6
  AND : Logic  IconShape=distinctive  AllPortsSameDT=off  OutDataTypeStr=boolean
  Add2 : Sum  OutDataTypeStr=Inherit: Same as first input
  Constant1 : Constant  Value=0  OutDataTypeStr=fixdt(0,rhoBits,0)  SampleTime=-1
  Multiport Switch{,1..3} (4 alike) : MultiPortSwitch  DataPortOrder=Zero-based contiguous  Inputs=2  zeroidx=on
  Relational Operator : RelationalOperator  Operator===  OutDataTypeStr=boolean  RndMeth=Simplest
  Simple Dual Port RAM : hdlsllib/HDL RAMs/Simple Dual Port RAM  ram_size=ceil(log2(rhoMax*2))
      settings: SourceProductBaseCode=SL
  Unit Delay{1..6} (6 alike) : UnitDelay  SampleTime=-1  HasFrameUpgradeWarning=on
  Hough Parameters : Outport
  wires:
  Valid/1 -> Multiport Switch/2
  Constant1/1 -> Multiport Switch2/3
  Unit Delay2/1 -> Relational Operator/1, Simple Dual Port RAM/2
  Unit Delay1/1 -> AND/1, Simple Dual Port RAM/3
  Rho/1 -> Multiport Switch1/2
  Clear/1 -> Multiport Switch/3
  Unit Delay3/1 -> Multiport Switch/1, Multiport Switch1/1, Multiport Switch2/1
  Multiport Switch2/1 -> Simple Dual Port RAM/1
  Multiport Switch/1 -> Unit Delay1/1
  Mode/1 -> Unit Delay3/1
  Address/1 -> Multiport Switch1/3
  Edge/1 -> Unit Delay4/1
  Multiport Switch1/1 -> Unit Delay2/1, Relational Operator/2, Simple Dual Port RAM/4
  Add2/1 -> Unit Delay5/1, Multiport Switch2/2
  Simple Dual Port RAM/1 -> Multiport Switch3/2, Hough Parameters/1
  Unit Delay5/1 -> Multiport Switch3/3
  AND/1 -> Unit Delay6/1
  Unit Delay6/1 -> Multiport Switch3/1
  Relational Operator/1 -> AND/2
  Multiport Switch3/1 -> Add2/1
  Unit Delay4/1 -> Add2/2
